simulink subsystem "subsistema_electrico_corriente_I_ds"  (R2023b)
settings: Solver=VariableStepAuto  StartTime=0.0  StopTime=10.0  RelTol=1e-3
values from neighbouring files (symbols this model uses):
  L_d = 6.6    [main.m]    (also in parametros.m = 0.0066)
  L_q = 5.8e-3    (= 0.0058)    [diagrama_polos_y_ceros_LTI.m]    (also in main.m = 5.8; parametros.m; variacion_de_parametros.m)
  P_p = 3    [diagrama_polos_y_ceros_LTI.m]    (also in main.m; parametros.m; variacion_de_parametros.m)
settings Model: Creator=nicol  LastModifiedBy=nicol

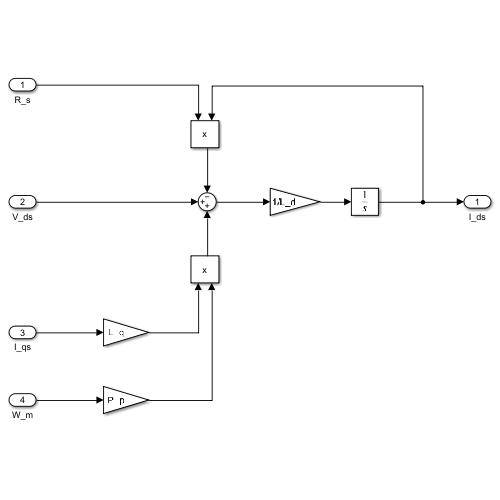
[thumbnail: Simulink's stored preview of the top-level diagram]
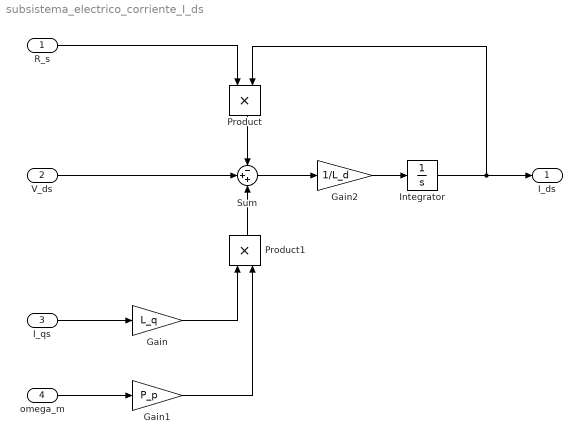
== system subsistema_electrico_corriente_I_ds ==
  R_s : Inport
  V_ds : Inport  Port=2
  I_qs : Inport  Port=3
  omega_m : Inport  Port=4
  Gain : Gain  Gain=L_q
  Gain1 : Gain  Gain=P_p
  Gain2 : Gain  Gain=1/L_d
  Integrator : Integrator
  Product : Product
  Product1 : Product
  Sum : Sum  Inputs=-++
  I_ds : Outport
  wires:
  R_s/1 -> Product/1
  V_ds/1 -> Sum/2
  I_qs/1 -> Gain/1
  Gain/1 -> Product1/1
  omega_m/1 -> Gain1/1
  Gain1/1 -> Product1/2
  Product1/1 -> Sum/3
  Product/1 -> Sum/1
  Sum/1 -> Gain2/1
  Gain2/1 -> Integrator/1
  Integrator/1 -> Product/2, I_ds/1
